simulink model "Bait_Ambrosino_kf"  (R2025b)
settings: Solver=VariableStepAuto  StartTime=0.0  StopTime=10.0  RelTol=1e-3
undefined symbols (not defined in the file): A, Akf, B, Bkf, C, Ckf, Dkf, K_lqi, nu, nx, ny, Qt, Rt, Ts, xref
libraries: simulink x2
settings Model: Creator=Miche  LastModifiedBy=Miche

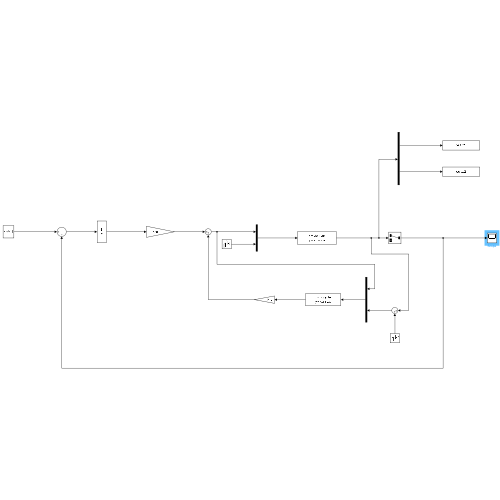
[thumbnail: Simulink's stored preview of the top-level diagram]
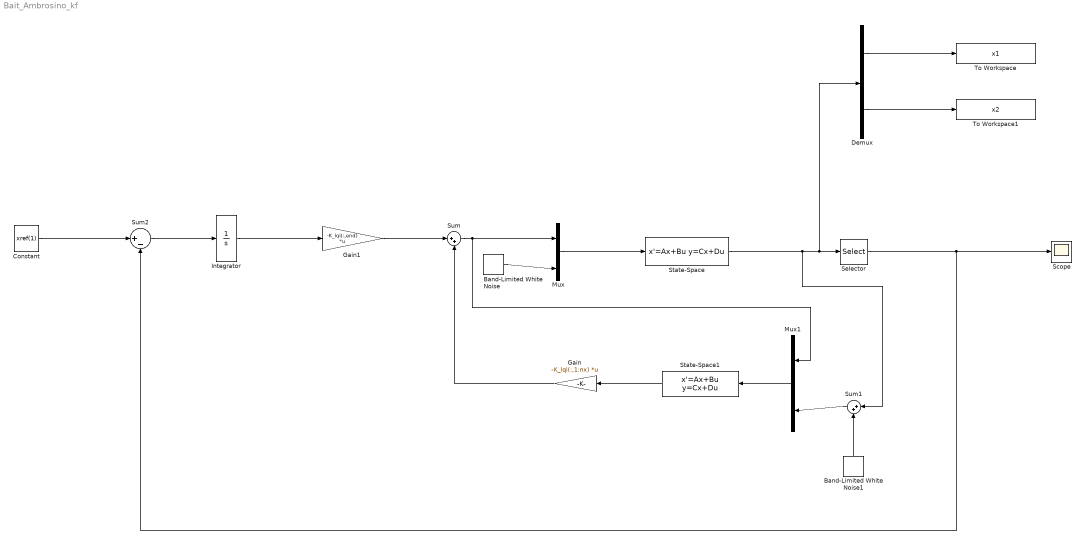
== system Bait_Ambrosino_kf ==
  Band-Limited White Noise : simulink/Sources/Band-Limited White Noise  Cov=diag(Qt)*Ts  Ts=Ts  seed=[23341]
  Band-Limited White Noise1 : simulink/Sources/Band-Limited White Noise  Cov=diag(Rt)*Ts  Ts=Ts  seed=[23341]
  Constant : Constant  Value=xref(1)
  Demux : Demux  Outputs=2
  Gain : Gain  Gain=-K_lqi(:,1:nx)  Multiplication=Matrix(K*u)
  Gain1 : Gain  Gain=-K_lqi(:,end)  Multiplication=Matrix(K*u)
  Integrator : Integrator
  Mux : Mux  Inputs=2
  Mux1 : Mux  Inputs=2
  Scope : Scope
      settings: ActiveDisplayYMinimum=-0.062642129612272182  ActiveDisplayYMaximum=0.56377916651044979
  Selector : Selector  InputPortWidth=2  IndexOptions=Index vector (dialog)  Indices=1  OutputSizes=1
  State-Space : StateSpace  A=A  B=[B eye(nx)]  C=C  D=zeros(ny,nu+nx)  InitialCondition=0
  State-Space1 : StateSpace  A=Akf  B=Bkf  C=Ckf  D=Dkf  InitialCondition=0
  Sum : Sum  Inputs=|++
  Sum1 : Sum  Inputs=|++
  Sum2 : Sum  Inputs=|+-
  To Workspace : ToWorkspace  VariableName=x1  SaveFormat=Timeseries  SampleTime=-1
  To Workspace1 : ToWorkspace  VariableName=x2  SaveFormat=Timeseries  SampleTime=-1
  wires:
  State-Space1/1 -> Gain/1
  Gain/1 -> Sum/2
  Sum/1 -> Mux1/1, Mux/1
  Band-Limited White Noise/1 -> Mux/2
  Mux/1 -> State-Space/1
  Mux1/1 -> State-Space1/1
  Band-Limited White Noise1/1 -> Sum1/2
  Sum1/1 -> Mux1/2
  Gain1/1 -> Sum/1
  Integrator/1 -> Gain1/1
  Selector/1 -> Sum2/2, Scope/1
  Sum2/1 -> Integrator/1
  Constant/1 -> Sum2/1
  Demux/2 -> To Workspace1/1
  State-Space/1 -> Sum1/1, Demux/1, Selector/1
  Demux/1 -> To Workspace/1
